simulink model "SPARCS_Mission_System_Composer"  (R2024a)
settings: Solver=VariableStepAuto  StartTime=0.0  StopTime=10.0  RelTol=1e-3
model workspace (MAT data in the model file):
  Communication_Data_Interface = Simulink.Bus
  Communication_Data_Interface.Alignment = -1
  Communication_Data_Interface.PreserveElementDimensions = 0
  Communication_Data_Interface.DataScope = 'Auto'
  Data_Interface = Simulink.Bus
  Data_Interface.Alignment = -1
  Data_Interface.PreserveElementDimensions = 0
  Data_Interface.DataScope = 'Auto'
  Mechanisem_Interface = Simulink.ConnectionBus
  Mechanisem_Interface.Elements_internal(1) = Simulink.ConnectionElement
  Mechanisem_Interface.Elements_internal(1).Name = 'Material'
  Mechanisem_Interface.Elements_internal(1).Type_internal = 'Connection: <domain name>'
  Mechanisem_Interface.Elements_internal(2) = Simulink.ConnectionElement
  Mechanisem_Interface.Elements_internal(2).Name = 'Inpute_Force'
  Mechanisem_Interface.Elements_internal(2).Type_internal = 'Connection: <domain name>'
  Power_Cable = Simulink.ConnectionBus
  Power_Cable.Elements_internal(1) = Simulink.ConnectionElement
  Power_Cable.Elements_internal(1).Name = 'v5'
  Power_Cable.Elements_internal(1).Type_internal = 'Connection: <domain name>'
  Power_Cable.Elements_internal(2) = Simulink.ConnectionElement
  Power_Cable.Elements_internal(2).Name = 'v33'
  Power_Cable.Elements_internal(2).Type_internal = 'Connection: <domain name>'
  Power_Cable.Elements_internal(3) = Simulink.ConnectionElement
  Power_Cable.Elements_internal(3).Name = 'v12'
  Power_Cable.Elements_internal(3).Type_internal = 'Connection: <domain name>'
  Power_Cable.Elements_internal(4) = Simulink.ConnectionElement
  Power_Cable.Elements_internal(4).Name = 'vUnreg'
  Power_Cable.Elements_internal(4).Type_internal = 'Connection: <domain name>'
  Power_Interface = Simulink.Bus
  Power_Interface.Alignment = -1
  Power_Interface.PreserveElementDimensions = 0
  Power_Interface.Elements_internal(1) = Simulink.BusElement
  Power_Interface.Elements_internal(1).Min_internal = 455
  Power_Interface.Elements_internal(1).DimensionsMode = 'Fixed'
  Power_Interface.Elements_internal(1).SamplingMode = 'Sample based'
  Power_Interface.Elements_internal(1).SampleTime = -1
  Power_Interface.Elements_internal(1).Name = 'InstCurrent'
  Power_Interface.Elements_internal(1).DataType_internal = 'double'
  Power_Interface.Elements_internal(1).Complexity = 'real'
  Power_Interface.Elements_internal(1).Dimensions = 1
  Power_Interface.Elements_internal(2) = Simulink.BusElement
  Power_Interface.Elements_internal(2).DimensionsMode = 'Fixed'
  Power_Interface.Elements_internal(2).SamplingMode = 'Sample based'
  Power_Interface.Elements_internal(2).SampleTime = -1
  Power_Interface.Elements_internal(2).Name = 'InstVoltage'
  Power_Interface.Elements_internal(2).DataType_internal = 'double'
  Power_Interface.Elements_internal(2).Complexity = 'real'
  Power_Interface.Elements_internal(2).Dimensions = 1
  Power_Interface.Elements_internal(3) = Simulink.BusElement
  Power_Interface.Elements_internal(3).DimensionsMode = 'Fixed'
  Power_Interface.Elements_internal(3).SamplingMode = 'Sample based'
  Power_Interface.Elements_internal(3).SampleTime = -1
  Power_Interface.Elements_internal(3).Name = 'BatteryVoltage'
  Power_Interface.Elements_internal(3).DataType_internal = 'double'
  Power_Interface.Elements_internal(3).Complexity = 'real'
  Power_Interface.Elements_internal(3).Dimensions = 1
  Power_Interface.DataScope = 'Auto'
undefined symbols (not defined in the file): ADCS, EPS, OBC, Power, TCS, Temp
(part 1 of 2)
settings Model: Creator=Mosavat  LastModifiedBy=dani
settings OptimizationCC: ReuseModelBlockBuffer=off
settings RTWCC: GPUComputeCapability=3.5

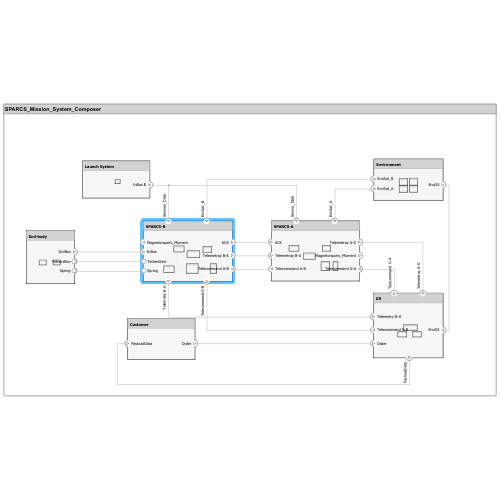
[thumbnail: Simulink's stored preview of the top-level diagram]
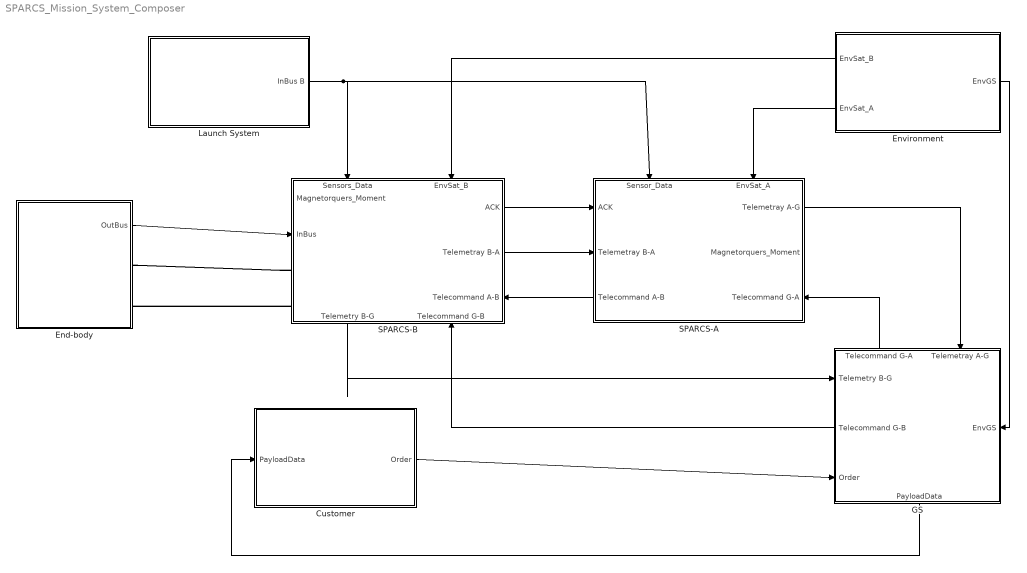
== system SPARCS_Mission_System_Composer ==
  Customer : Subsystem  RequirementInfo={} %GIDa_5276cd9e_2c2d_434b_852c_f5458c074aea
      settings: PortSchema="{\"entries\":[{\"content\":{\"headerSize\":26,\"margin\":15,\"minimumSpacing\":25,\"sides\":[{\"content\":{\"connectorIds\":[\"In1\"]},\"type\":\"ConnectorPlacement.EquallySpacedRectSide\",\"uuid\":\"99c16914-1f21-4030-bd23-0dca739cb4ef\"},{\"content\":{\"connectorIds\":[\"Out1\"],\"side\":\"RIGHT\"},\"type\":\"ConnectorPlacement.EquallySpacedRectSide\",\"uuid\":\"ee0d90fc-8c9e-49ed-bf7b-51fc360639f9\"},{\"content\":{\"connectorIds\":[],\"side\":\"TOP\"},\"type\":\"ConnectorPlacement.EquallySpacedRectSide\",\"uuid\":\"43e54e8f-1cc4-498f-b673-46655361aaba\"}]},\"type\":\"ConnectorPlacement.EquallySpacedConnector\",\"uuid\":\"2a460a3b-dd2b-4c63-a476-f56c55e2bff6\"}],\"packageUris\":[\"http://schema.mathworks.com/mf0/Connector/R2020b\"],\"version\":\"1.0\"}"
  End-body : Subsystem
      settings: PortSchema="{\"entries\":[{\"content\":{\"headerSize\":26,\"margin\":15,\"minimumSpacing\":25,\"sides\":[{\"content\":{\"connectorIds\":[]},\"type\":\"ConnectorPlacement.EquallySpacedRectSide\",\"uuid\":\"e9a48b2f-fbc4-402d-8d97-df232b09ca74\"},{\"content\":{\"connectorIds\":[\"Out1\",\"RConn1\",\"RConn2\"],\"side\":\"RIGHT\"},\"type\":\"ConnectorPlacement.EquallySpacedRectSide\",\"uuid\":\"668a9a5e-c59a-482e-88a8-af4c8ec5a9f3\"},{\"content\":{\"connectorIds\":[],\"side\":\"TOP\"},\"type\":\"ConnectorPlacement.EquallySpacedRectSide\",\"uuid\":\"7c7fce8b-f648-49b4-9dc1-b61d0240baf7\"}]},\"type\":\"ConnectorPlacement.EquallySpacedConnector\",\"uuid\":\"1f193ebe-c506-4262-ad28-c863fe0100e9\"}],\"packageUris\":[\"http://schema.mathworks.com/mf0/Connector/R2020b\"],\"version\":\"1.0\"}"
  Environment : Subsystem  RequirementInfo={} %GIDa_2c95b2b7_b51e_4aa9_866b_417deecfb3d4
      settings: PortSchema="{\"entries\":[{\"content\":{\"headerSize\":26,\"margin\":15,\"minimumSpacing\":25,\"sides\":[{\"content\":{\"connectorIds\":[\"Out1\",\"Out3\"]},\"type\":\"ConnectorPlacement.EquallySpacedRectSide\",\"uuid\":\"99c16914-1f21-4030-bd23-0dca739cb4ef\"},{\"content\":{\"connectorIds\":[\"Out2\"],\"side\":\"RIGHT\"},\"type\":\"ConnectorPlacement.EquallySpacedRectSide\",\"uuid\":\"ee0d90fc-8c9e-49ed-bf7b-51fc360639f9\"},{\"content\":{\"side\":\"TOP\"},\"type\":\"ConnectorPlacement.EquallySpacedRectSide\",\"uuid\":\"43e54e8f-1cc4-498f-b673-46655361aaba\"},{\"content\":{\"side\":\"BOTTOM\"},\"type\":\"ConnectorPlacement.EquallySpacedRectSide\",\"uuid\":\"c295d207-1cb1-4ab0-ab4a-221cf9a33f8c\"}]},\"type\":\"ConnectorPlacement.EquallySpacedConnector\",\"uuid\":\"2a460a3b-dd2b-4c63-a476-f56c55e2bff6\"}],\"packageUris\":[\"http://schema.mathworks.com/mf0/Connector/R2020b\"],\"version\":\"1.0\"}"
  GS : Subsystem  RequirementInfo={} %GIDa_7f442463_82d1_4b26_b178_1c38fd973034
      settings: PortSchema="{\"entries\":[{\"content\":{\"headerSize\":26,\"margin\":15,\"minimumSpacing\":25,\"sides\":[{\"content\":{\"connectorIds\":[\"In1\",\"Out1\",\"In2\"]},\"type\":\"ConnectorPlacement.EquallySpacedRectSide\",\"uuid\":\"99c16914-1f21-4030-bd23-0dca739cb4ef\"},{\"content\":{\"connectorIds\":[\"In4\"],\"side\":\"RIGHT\"},\"type\":\"ConnectorPlacement.EquallySpacedRectSide\",\"uuid\":\"ee0d90fc-8c9e-49ed-bf7b-51fc360639f9\"},{\"content\":{\"connectorIds\":[\"Out3\",\"In3\"],\"side\":\"TOP\"},\"type\":\"ConnectorPlacement.EquallySpacedRectSide\",\"uuid\":\"43e54e8f-1cc4-498f-b673-46655361aaba\"},{\"content\":{\"connectorIds\":[\"Out2\"],\"side\":\"BOTTOM\"},\"type\":\"ConnectorPlacement.EquallySpacedRectSide\",\"uuid\":\"61113e39-adc5-4e36-8ba9-18f5b15ab978\"}]},\"type\":\"ConnectorPlacement.EquallySpacedConnector\",\"uuid\":\"2a460a3b-dd2b-4c63-a476-f56c55e2bff6\"}],\"packageUris\":[\"http://schema.mathworks.com/mf0/Connector/R2020b\"],\"version\":\"1.0\"}"
  Launch System : Subsystem  RequirementInfo={} %GIDa_9d5cdb3d_6dc4_4d26_bfc5_e8ae113977f2
      settings: PortSchema="{\"entries\":[{\"content\":{\"headerSize\":26,\"margin\":15,\"minimumSpacing\":25,\"sides\":[{\"content\":{\"connectorIds\":[]},\"type\":\"ConnectorPlacement.EquallySpacedRectSide\",\"uuid\":\"0e80917e-0df8-41c9-b4a1-578069d1b510\"},{\"content\":{\"connectorIds\":[\"Out1\"],\"side\":\"RIGHT\"},\"type\":\"ConnectorPlacement.EquallySpacedRectSide\",\"uuid\":\"65f7606d-47df-4668-9c7a-3f7124642eb8\"},{\"content\":{\"connectorIds\":[],\"side\":\"TOP\"},\"type\":\"ConnectorPlacement.EquallySpacedRectSide\",\"uuid\":\"3548d248-01fd-4db2-a2f6-b603deefc062\"}]},\"type\":\"ConnectorPlacement.EquallySpacedConnector\",\"uuid\":\"f365137c-e6cc-4032-bc65-cfd89a070f7f\"}],\"packageUris\":[\"http://schema.mathworks.com/mf0/Connector/R2020b\"],\"version\":\"1.0\"}"
  SPARCS-A : Subsystem  RequirementInfo="{}  %GIDa_bb889290_f2af_4178_93e4_6d667fc14114"
      settings: PortSchema="{\"entries\":[{\"content\":{\"headerSize\":26,\"margin\":15,\"minimumSpacing\":25,\"sides\":[{\"content\":{\"connectorIds\":[\"In1\",\"In2\",\"Out1\"]},\"type\":\"ConnectorPlacement.EquallySpacedRectSide\",\"uuid\":\"e9a48b2f-fbc4-402d-8d97-df232b09ca74\"},{\"content\":{\"connectorIds\":[\"Out3\",\"Out2\",\"In3\"],\"side\":\"RIGHT\"},\"type\":\"ConnectorPlacement.EquallySpacedRectSide\",\"uuid\":\"668a9a5e-c59a-482e-88a8-af4c8ec5a9f3\"},{\"content\":{\"connectorIds\":[\"In4\",\"In5\"],\"side\":\"TOP\"},\"type\":\"ConnectorPlacement.EquallySpacedRectSide\",\"uuid\":\"7c7fce8b-f648-49b4-9dc1-b61d0240baf7\"}]},\"type\":\"ConnectorPlacement.EquallySpacedConnector\",\"uuid\":\"1f193ebe-c506-4262-ad28-c863fe0100e9\"}],\"packageUris\":[\"http://schema.mathworks.com/mf0/Connector/R2020b\"],\"version\":\"1.0\"}"
  SPARCS-B : Subsystem
      settings: PortSchema="{\"entries\":[{\"content\":{\"headerSize\":26,\"margin\":15,\"minimumSpacing\":25,\"sides\":[{\"content\":{\"connectorIds\":[\"Out3\",\"In3\",\"LConn1\",\"LConn2\"]},\"type\":\"ConnectorPlacement.EquallySpacedRectSide\",\"uuid\":\"e9a48b2f-fbc4-402d-8d97-df232b09ca74\"},{\"content\":{\"connectorIds\":[\"Out2\",\"Out4\",\"In4\"],\"side\":\"RIGHT\"},\"type\":\"ConnectorPlacement.EquallySpacedRectSide\",\"uuid\":\"668a9a5e-c59a-482e-88a8-af4c8ec5a9f3\"},{\"content\":{\"connectorIds\":[\"In5\",\"In2\"],\"side\":\"TOP\"},\"type\":\"ConnectorPlacement.EquallySpacedRectSide\",\"uuid\":\"7c7fce8b-f648-49b4-9dc1-b61d0240baf7\"},{\"content\":{\"connectorIds\":[\"Out1\",\"In1\"],\"side\":\"BOTTOM\"},\"type\":\"ConnectorPlacement.EquallySpacedRectSide\",\"uuid\":\"24f8add0-5994-41fc-ad83-a43d4515e3f5\"}]},\"type\":\"ConnectorPlacement.EquallySpacedConnector\",\"uuid\":\"1f193ebe-c506-4262-ad28-c863fe0100e9\"}],\"packageUris\":[\"http://schema.mathworks.com/mf0/Connector/R2020b\"],\"version\":\"1.0\"}"
  wires:
  Launch System/1(InBus B) -> SPARCS-A/4(Sensor_Data), SPARCS-B/5(Sensors_Data)
  Environment/3(EnvSat_A) -> SPARCS-A/5(EnvSat_A)
  Environment/2(EnvGS) -> GS/4(EnvGS)
  GS/3(Telecommand G-A) -> SPARCS-A/3(Telecommand G-A)
  SPARCS-A/3(Telemetray A-G) -> GS/3(Telemetray A-G)
  Customer/1(Order) -> GS/2(Order)
  GS/2(PayloadData) -> Customer/1(PayloadData)
  SPARCS-B/4(Telemetray B-A) -> SPARCS-A/2(Telemetray B-A)
  SPARCS-A/1(Telecommand A-B) -> SPARCS-B/4(Telecommand A-B)
  End-body/1(OutBus) -> SPARCS-B/3(InBus)
  SPARCS-B/2(ACK) -> SPARCS-A/1(ACK)
  SPARCS-B/1(Telemetry B-G) -> GS/1(Telemetry B-G)
  GS/1(Telecommand G-B) -> SPARCS-B/1(Telecommand G-B)
  Environment/1(EnvSat_B) -> SPARCS-B/2(EnvSat_B)
  connections:
  SPARCS-B/LConn1 -- End-body/RConn1
  SPARCS-B/LConn2 -- End-body/RConn2

== system SPARCS_Mission_System_Composer/Customer ==
  Bus Element In1 : Inport  RequirementInfo={} %GIDa_50217abe_56c4_45ce_a731_87f8e4f342ac  PortName=PayloadData
  Bus Element Out1 : Outport  RequirementInfo={} %GIDa_63cfd474_b787_456e_9731_ad5e1ed17cae  PortName=Order

== system SPARCS_Mission_System_Composer/End-body ==
  Collector : Subsystem
      settings: PortSchema="{\"entries\":[{\"content\":{\"headerSize\":26,\"margin\":15,\"minimumSpacing\":25,\"sides\":[{\"content\":{\"connectorIds\":[]},\"type\":\"ConnectorPlacement.EquallySpacedRectSide\",\"uuid\":\"b0f3186e-f576-4647-b1a2-44485358b727\"},{\"content\":{\"connectorIds\":[],\"side\":\"RIGHT\"},\"type\":\"ConnectorPlacement.EquallySpacedRectSide\",\"uuid\":\"71064ded-3aa0-4a06-beed-3d1d2c210288\"},{\"content\":{\"connectorIds\":[],\"side\":\"TOP\"},\"type\":\"ConnectorPlacement.EquallySpacedRectSide\",\"uuid\":\"7b8a25e8-1259-40c4-b5f8-7d1b8fa69d47\"}]},\"type\":\"ConnectorPlacement.EquallySpacedConnector\",\"uuid\":\"e60708fb-7212-4361-80b1-30af05aaea9b\"}],\"packageUris\":[\"http://schema.mathworks.com/mf0/Connector/R2020b\"],\"version\":\"1.0\"}"
  Emitter : Subsystem
      settings: PortSchema="{\"entries\":[{\"content\":{\"headerSize\":26,\"margin\":15,\"minimumSpacing\":25,\"sides\":[{\"content\":{\"connectorIds\":[]},\"type\":\"ConnectorPlacement.EquallySpacedRectSide\",\"uuid\":\"b0f3186e-f576-4647-b1a2-44485358b727\"},{\"content\":{\"connectorIds\":[],\"side\":\"RIGHT\"},\"type\":\"ConnectorPlacement.EquallySpacedRectSide\",\"uuid\":\"71064ded-3aa0-4a06-beed-3d1d2c210288\"},{\"content\":{\"connectorIds\":[],\"side\":\"TOP\"},\"type\":\"ConnectorPlacement.EquallySpacedRectSide\",\"uuid\":\"7b8a25e8-1259-40c4-b5f8-7d1b8fa69d47\"}]},\"type\":\"ConnectorPlacement.EquallySpacedConnector\",\"uuid\":\"e60708fb-7212-4361-80b1-30af05aaea9b\"}],\"packageUris\":[\"http://schema.mathworks.com/mf0/Connector/R2020b\"],\"version\":\"1.0\"}"
  TetherWire : PMIOPort  Side=Right
  Spring : PMIOPort  Port=2  Side=Right
  Bus Element Out1 : Outport  PortName=OutBus

== system SPARCS_Mission_System_Composer/Environment ==
  Atmosphere : Subsystem  RequirementInfo={} %GIDa_eb05b99d_c241_4e54_a779_761c9347d3e2
      settings: PortSchema="{\"entries\":[{\"content\":{\"headerSize\":26,\"margin\":15,\"minimumSpacing\":25,\"sides\":[{\"content\":{\"connectorIds\":[]},\"type\":\"ConnectorPlacement.EquallySpacedRectSide\",\"uuid\":\"a0205618-f388-4a93-9aec-aa689e4ebd78\"},{\"content\":{\"connectorIds\":[],\"side\":\"RIGHT\"},\"type\":\"ConnectorPlacement.EquallySpacedRectSide\",\"uuid\":\"79acb52b-c683-45c4-8f19-6aa7b44b6a95\"},{\"content\":{\"connectorIds\":[],\"side\":\"TOP\"},\"type\":\"ConnectorPlacement.EquallySpacedRectSide\",\"uuid\":\"1a3a54da-b4f5-4a0e-9102-49590a789f5c\"}]},\"type\":\"ConnectorPlacement.EquallySpacedConnector\",\"uuid\":\"e5b731ae-b390-48dd-b7a1-3459e2e6bab0\"}],\"packageUris\":[\"http://schema.mathworks.com/mf0/Connector/R2020b\"],\"version\":\"1.0\"}"
  Earth : Subsystem  RequirementInfo={} %GIDa_b95c931a_ef81_4893_b6c0_be75a463d49e
      settings: PortSchema="{\"entries\":[{\"content\":{\"headerSize\":26,\"margin\":15,\"minimumSpacing\":25,\"sides\":[{\"content\":{\"connectorIds\":[]},\"type\":\"ConnectorPlacement.EquallySpacedRectSide\",\"uuid\":\"a0205618-f388-4a93-9aec-aa689e4ebd78\"},{\"content\":{\"connectorIds\":[],\"side\":\"RIGHT\"},\"type\":\"ConnectorPlacement.EquallySpacedRectSide\",\"uuid\":\"79acb52b-c683-45c4-8f19-6aa7b44b6a95\"},{\"content\":{\"connectorIds\":[],\"side\":\"TOP\"},\"type\":\"ConnectorPlacement.EquallySpacedRectSide\",\"uuid\":\"1a3a54da-b4f5-4a0e-9102-49590a789f5c\"}]},\"type\":\"ConnectorPlacement.EquallySpacedConnector\",\"uuid\":\"e5b731ae-b390-48dd-b7a1-3459e2e6bab0\"}],\"packageUris\":[\"http://schema.mathworks.com/mf0/Connector/R2020b\"],\"version\":\"1.0\"}"
  Sun : Subsystem  RequirementInfo={} %GIDa_99381c14_de20_4199_bf05_b451084bd8b9
      settings: PortSchema="{\"entries\":[{\"content\":{\"headerSize\":26,\"margin\":15,\"minimumSpacing\":25,\"sides\":[{\"content\":{\"connectorIds\":[]},\"type\":\"ConnectorPlacement.EquallySpacedRectSide\",\"uuid\":\"a0205618-f388-4a93-9aec-aa689e4ebd78\"},{\"content\":{\"connectorIds\":[],\"side\":\"RIGHT\"},\"type\":\"ConnectorPlacement.EquallySpacedRectSide\",\"uuid\":\"79acb52b-c683-45c4-8f19-6aa7b44b6a95\"},{\"content\":{\"connectorIds\":[],\"side\":\"TOP\"},\"type\":\"ConnectorPlacement.EquallySpacedRectSide\",\"uuid\":\"1a3a54da-b4f5-4a0e-9102-49590a789f5c\"}]},\"type\":\"ConnectorPlacement.EquallySpacedConnector\",\"uuid\":\"e5b731ae-b390-48dd-b7a1-3459e2e6bab0\"}],\"packageUris\":[\"http://schema.mathworks.com/mf0/Connector/R2020b\"],\"version\":\"1.0\"}"
  Time : Subsystem  RequirementInfo={} %GIDa_8bde8406_355b_4db9_a468_32211b2e0ea2
      settings: PortSchema="{\"entries\":[{\"content\":{\"headerSize\":26,\"margin\":15,\"minimumSpacing\":25,\"sides\":[{\"content\":{\"connectorIds\":[]},\"type\":\"ConnectorPlacement.EquallySpacedRectSide\",\"uuid\":\"a0205618-f388-4a93-9aec-aa689e4ebd78\"},{\"content\":{\"connectorIds\":[],\"side\":\"RIGHT\"},\"type\":\"ConnectorPlacement.EquallySpacedRectSide\",\"uuid\":\"79acb52b-c683-45c4-8f19-6aa7b44b6a95\"},{\"content\":{\"connectorIds\":[],\"side\":\"TOP\"},\"type\":\"ConnectorPlacement.EquallySpacedRectSide\",\"uuid\":\"1a3a54da-b4f5-4a0e-9102-49590a789f5c\"}]},\"type\":\"ConnectorPlacement.EquallySpacedConnector\",\"uuid\":\"e5b731ae-b390-48dd-b7a1-3459e2e6bab0\"}],\"packageUris\":[\"http://schema.mathworks.com/mf0/Connector/R2020b\"],\"version\":\"1.0\"}"
  Bus Element Out3 : Outport  PortName=EnvSat_B
  Bus Element Out2 : Outport  RequirementInfo={} %GIDa_4f6e6d30_9ff6_4620_aadf_7d15cb6fc292  Port=2  PortName=EnvGS
  Bus Element Out1 : Outport  RequirementInfo={} %GIDa_ad4902e5_7a7f_4265_b3dc_3808822d8108  Port=3  PortName=EnvSat_A

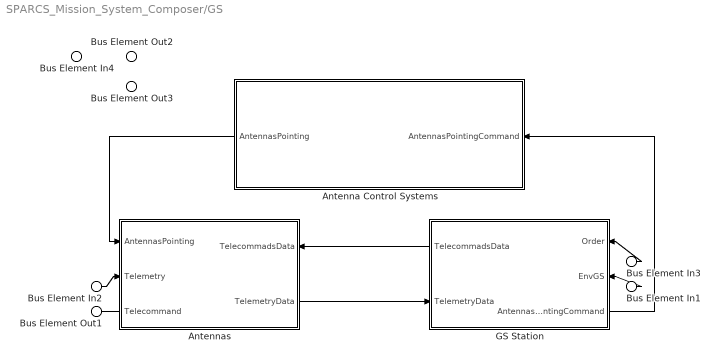
== system SPARCS_Mission_System_Composer/GS ==
  Bus Element In4 : Inport  PortName=Telemetry B-G
  Bus Element In3 : Inport  RequirementInfo={} %GIDa_1c5e6e98_e2f6_49b9_9cfa_88040fc1fba5  Port=2  PortName=Order
  Bus Element In2 : Inport  RequirementInfo={} %GIDa_0c79b00d_9eca_49d8_adcc_d17375f08e84  Port=3  PortName=Telemetray A-G
  Bus Element In1 : Inport  RequirementInfo={} %GIDa_ac8f2bba_56c0_4e78_a408_5eec346da907  Port=4  PortName=EnvGS
  Antenna Control Systems : Subsystem  RequirementInfo={} %GIDa_89f6fcc8_7c51_47bb_b8d5_8a1504126ec7
      settings: PortSchema="{\"entries\":[{\"content\":{\"headerSize\":26,\"margin\":15,\"minimumSpacing\":25,\"sides\":[{\"content\":{\"connectorIds\":[\"Out1\"]},\"type\":\"ConnectorPlacement.EquallySpacedRectSide\",\"uuid\":\"a0205618-f388-4a93-9aec-aa689e4ebd78\"},{\"content\":{\"connectorIds\":[\"In1\"],\"side\":\"RIGHT\"},\"type\":\"ConnectorPlacement.EquallySpacedRectSide\",\"uuid\":\"79acb52b-c683-45c4-8f19-6aa7b44b6a95\"},{\"content\":{\"connectorIds\":[],\"side\":\"TOP\"},\"type\":\"ConnectorPlacement.EquallySpacedRectSide\",\"uuid\":\"1a3a54da-b4f5-4a0e-9102-49590a789f5c\"},{\"content\":{\"connectorIds\":[],\"side\":\"BOTTOM\"},\"type\":\"ConnectorPlacement.EquallySpacedRectSide\",\"uuid\":\"9ac2cda3-0247-4f52-b572-2154d037acfc\"}]},\"type\":\"ConnectorPlacement.EquallySpacedConnector\",\"uuid\":\"e5b731ae-b390-48dd-b7a1-3459e2e6bab0\"}],\"packageUris\":[\"http://schema.mathworks.com/mf0/Connector/R2020b\"],\"version\":\"1.0\"}"
  Antennas : Subsystem  RequirementInfo={} %GIDa_95957288_8d11_42dc_b667_82305f244e57
      settings: PortSchema="{\"entries\":[{\"content\":{\"headerSize\":26,\"margin\":15,\"minimumSpacing\":25,\"sides\":[{\"content\":{\"connectorIds\":[\"In2\",\"In3\",\"Out2\"]},\"type\":\"ConnectorPlacement.EquallySpacedRectSide\",\"uuid\":\"a0205618-f388-4a93-9aec-aa689e4ebd78\"},{\"content\":{\"connectorIds\":[\"In1\",\"Out1\"],\"side\":\"RIGHT\"},\"type\":\"ConnectorPlacement.EquallySpacedRectSide\",\"uuid\":\"79acb52b-c683-45c4-8f19-6aa7b44b6a95\"},{\"content\":{\"connectorIds\":[],\"side\":\"TOP\"},\"type\":\"ConnectorPlacement.EquallySpacedRectSide\",\"uuid\":\"1a3a54da-b4f5-4a0e-9102-49590a789f5c\"}]},\"type\":\"ConnectorPlacement.EquallySpacedConnector\",\"uuid\":\"e5b731ae-b390-48dd-b7a1-3459e2e6bab0\"}],\"packageUris\":[\"http://schema.mathworks.com/mf0/Connector/R2020b\"],\"version\":\"1.0\"}"
  GS Station : Subsystem  RequirementInfo={} %GIDa_50bc68e1_b1a0_408f_93ec_e9ab810c3ebe
      settings: PortSchema="{\"entries\":[{\"content\":{\"headerSize\":26,\"margin\":15,\"minimumSpacing\":25,\"sides\":[{\"content\":{\"connectorIds\":[\"Out1\",\"In3\"]},\"type\":\"ConnectorPlacement.EquallySpacedRectSide\",\"uuid\":\"a0205618-f388-4a93-9aec-aa689e4ebd78\"},{\"content\":{\"connectorIds\":[\"In1\",\"In2\",\"Out2\"],\"side\":\"RIGHT\"},\"type\":\"ConnectorPlacement.EquallySpacedRectSide\",\"uuid\":\"79acb52b-c683-45c4-8f19-6aa7b44b6a95\"},{\"content\":{\"connectorIds\":[],\"side\":\"TOP\"},\"type\":\"ConnectorPlacement.EquallySpacedRectSide\",\"uuid\":\"1a3a54da-b4f5-4a0e-9102-49590a789f5c\"},{\"content\":{\"connectorIds\":[],\"side\":\"BOTTOM\"},\"type\":\"ConnectorPlacement.EquallySpacedRectSide\",\"uuid\":\"a0883a5f-cb12-4437-b239-442920e299fa\"}]},\"type\":\"ConnectorPlacement.EquallySpacedConnector\",\"uuid\":\"e5b731ae-b390-48dd-b7a1-3459e2e6bab0\"}],\"packageUris\":[\"http://schema.mathworks.com/mf0/Connector/R2020b\"],\"version\":\"1.0\"}"
  Bus Element Out3 : Outport  PortName=Telecommand G-B
  Bus Element Out2 : Outport  Port=2  PortName=PayloadData
  Bus Element Out1 : Outport  RequirementInfo={} %GIDa_51763359_9ab6_48ad_b447_d543d03ee004  Port=3  PortName=Telecommand G-A
  wires:
  Bus Element In2/1 -> Antennas/3(Telemetry)
  Antennas/2(Telecommand) -> Bus Element Out1/1
  Antenna Control Systems/1(AntennasPointing) -> Antennas/2(AntennasPointing)
  GS Station/2(AntennasPointingCommand) -> Antenna Control Systems/1(AntennasPointingCommand)
  GS Station/1(TelecommadsData) -> Antennas/1(TelecommadsData)
  Antennas/1(TelemetryData) -> GS Station/3(TelemetryData)
  Bus Element In1/1 -> GS Station/2(EnvGS)
  Bus Element In3/1 -> GS Station/1(Order)

== system SPARCS_Mission_System_Composer/Launch System ==
  Component : Subsystem
      settings: PortSchema="{\"entries\":[{\"content\":{\"headerSize\":26,\"margin\":15,\"minimumSpacing\":25,\"sides\":[{\"content\":{\"connectorIds\":[]},\"type\":\"ConnectorPlacement.EquallySpacedRectSide\",\"uuid\":\"9a7037ce-e1a5-4d46-8111-5886fddb9b24\"},{\"content\":{\"connectorIds\":[],\"side\":\"RIGHT\"},\"type\":\"ConnectorPlacement.EquallySpacedRectSide\",\"uuid\":\"20b2048c-0904-414d-8c49-ea2b529604ef\"},{\"content\":{\"connectorIds\":[],\"side\":\"TOP\"},\"type\":\"ConnectorPlacement.EquallySpacedRectSide\",\"uuid\":\"32c6da6e-71f7-4ed5-82cb-cf1b28c2bdf7\"}]},\"type\":\"ConnectorPlacement.EquallySpacedConnector\",\"uuid\":\"f6c8ad2c-3d58-4ab6-b863-3f028749c78d\"}],\"packageUris\":[\"http://schema.mathworks.com/mf0/Connector/R2020b\"],\"version\":\"1.0\"}"
  Bus Element Out1 : Outport  RequirementInfo={} %GIDa_f2808e3f_afc6_412a_b6c0_e64b71cecebd  PortName=InBus B

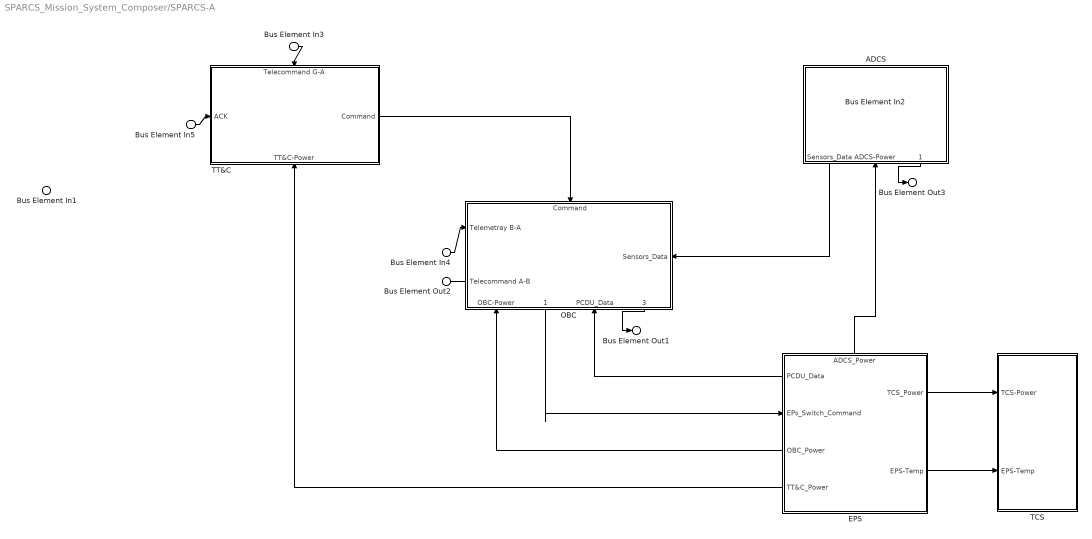
== system SPARCS_Mission_System_Composer/SPARCS-A ==
  Bus Element In5 : Inport  PortName=ACK
  Bus Element In4 : Inport  Port=2  PortName=Telemetray B-A
  Bus Element In3 : Inport  Port=3  PortName=Telecommand G-A
  Bus Element In1 : Inport  Port=4  PortName=Sensor_Data
  Bus Element In2 : Inport  Port=5  PortName=EnvSat_A
  ADCS : Subsystem
      settings: PortSchema="{\"entries\":[{\"content\":{\"headerSize\":26,\"margin\":15,\"minimumSpacing\":25,\"sides\":[{\"content\":{\"connectorIds\":[]},\"type\":\"ConnectorPlacement.EquallySpacedRectSide\",\"uuid\":\"e9a48b2f-fbc4-402d-8d97-df232b09ca74\"},{\"content\":{\"connectorIds\":[],\"side\":\"RIGHT\"},\"type\":\"ConnectorPlacement.EquallySpacedRectSide\",\"uuid\":\"668a9a5e-c59a-482e-88a8-af4c8ec5a9f3\"},{\"content\":{\"connectorIds\":[],\"side\":\"TOP\"},\"type\":\"ConnectorPlacement.EquallySpacedRectSide\",\"uuid\":\"7c7fce8b-f648-49b4-9dc1-b61d0240baf7\"},{\"content\":{\"connectorIds\":[\"Out2\",\"In1\",\"Out1\"],\"side\":\"BOTTOM\"},\"type\":\"ConnectorPlacement.EquallySpacedRectSide\",\"uuid\":\"2c3f5986-9b39-4ef3-b054-4f041a587ca4\"}]},\"type\":\"ConnectorPlacement.EquallySpacedConnector\",\"uuid\":\"1f193ebe-c506-4262-ad28-c863fe0100e9\"}],\"packageUris\":[\"http://schema.mathworks.com/mf0/Connector/R2020b\"],\"version\":\"1.0\"}"
  EPS : Subsystem
      settings: PortSchema="{\"entries\":[{\"content\":{\"headerSize\":26,\"margin\":15,\"minimumSpacing\":25,\"sides\":[{\"content\":{\"connectorIds\":[\"Out1\",\"In1\",\"Out5\",\"Out6\"]},\"type\":\"ConnectorPlacement.EquallySpacedRectSide\",\"uuid\":\"e9a48b2f-fbc4-402d-8d97-df232b09ca74\"},{\"content\":{\"connectorIds\":[\"Out2\",\"Out3\"],\"side\":\"RIGHT\"},\"type\":\"ConnectorPlacement.EquallySpacedRectSide\",\"uuid\":\"668a9a5e-c59a-482e-88a8-af4c8ec5a9f3\"},{\"content\":{\"connectorIds\":[\"Out4\"],\"side\":\"TOP\"},\"type\":\"ConnectorPlacement.EquallySpacedRectSide\",\"uuid\":\"7c7fce8b-f648-49b4-9dc1-b61d0240baf7\"},{\"content\":{\"connectorIds\":[],\"side\":\"BOTTOM\"},\"type\":\"ConnectorPlacement.EquallySpacedRectSide\",\"uuid\":\"3e521869-eeda-4ec5-bb7d-2b348f8e7054\"}]},\"type\":\"ConnectorPlacement.EquallySpacedConnector\",\"uuid\":\"1f193ebe-c506-4262-ad28-c863fe0100e9\"}],\"packageUris\":[\"http://schema.mathworks.com/mf0/Connector/R2020b\"],\"version\":\"1.0\"}"
  OBC : Subsystem
      settings: PortSchema="{\"entries\":[{\"content\":{\"headerSize\":26,\"margin\":15,\"minimumSpacing\":25,\"sides\":[{\"content\":{\"connectorIds\":[\"In3\",\"Out2\"]},\"type\":\"ConnectorPlacement.EquallySpacedRectSide\",\"uuid\":\"e9a48b2f-fbc4-402d-8d97-df232b09ca74\"},{\"content\":{\"connectorIds\":[\"In4\"],\"side\":\"RIGHT\"},\"type\":\"ConnectorPlacement.EquallySpacedRectSide\",\"uuid\":\"668a9a5e-c59a-482e-88a8-af4c8ec5a9f3\"},{\"content\":{\"connectorIds\":[\"In1\"],\"side\":\"TOP\"},\"type\":\"ConnectorPlacement.EquallySpacedRectSide\",\"uuid\":\"7c7fce8b-f648-49b4-9dc1-b61d0240baf7\"},{\"content\":{\"connectorIds\":[\"In5\",\"Out1\",\"In2\",\"Out3\"],\"side\":\"BOTTOM\"},\"type\":\"ConnectorPlacement.EquallySpacedRectSide\",\"uuid\":\"b1c700a7-d344-470e-b338-9b978c458512\"}]},\"type\":\"ConnectorPlacement.EquallySpacedConnector\",\"uuid\":\"1f193ebe-c506-4262-ad28-c863fe0100e9\"}],\"packageUris\":[\"http://schema.mathworks.com/mf0/Connector/R2020b\"],\"version\":\"1.0\"}"
  TCS : Subsystem
      settings: PortSchema="{\"entries\":[{\"content\":{\"headerSize\":26,\"margin\":15,\"minimumSpacing\":25,\"sides\":[{\"content\":{\"connectorIds\":[\"In2\",\"In1\"]},\"type\":\"ConnectorPlacement.EquallySpacedRectSide\",\"uuid\":\"e9a48b2f-fbc4-402d-8d97-df232b09ca74\"},{\"content\":{\"connectorIds\":[],\"side\":\"RIGHT\"},\"type\":\"ConnectorPlacement.EquallySpacedRectSide\",\"uuid\":\"668a9a5e-c59a-482e-88a8-af4c8ec5a9f3\"},{\"content\":{\"connectorIds\":[],\"side\":\"TOP\"},\"type\":\"ConnectorPlacement.EquallySpacedRectSide\",\"uuid\":\"7c7fce8b-f648-49b4-9dc1-b61d0240baf7\"},{\"content\":{\"connectorIds\":[],\"side\":\"BOTTOM\"},\"type\":\"ConnectorPlacement.EquallySpacedRectSide\",\"uuid\":\"b0f76e66-ab31-4e75-aed3-a16376b57c27\"}]},\"type\":\"ConnectorPlacement.EquallySpacedConnector\",\"uuid\":\"1f193ebe-c506-4262-ad28-c863fe0100e9\"}],\"packageUris\":[\"http://schema.mathworks.com/mf0/Connector/R2020b\"],\"version\":\"1.0\"}"
  "TT&C " : Subsystem
      settings: PortSchema="{\"entries\":[{\"content\":{\"headerSize\":26,\"margin\":15,\"minimumSpacing\":25,\"sides\":[{\"content\":{\"connectorIds\":[\"In1\"]},\"type\":\"ConnectorPlacement.EquallySpacedRectSide\",\"uuid\":\"e9a48b2f-fbc4-402d-8d97-df232b09ca74\"},{\"content\":{\"connectorIds\":[\"Out1\"],\"side\":\"RIGHT\"},\"type\":\"ConnectorPlacement.EquallySpacedRectSide\",\"uuid\":\"668a9a5e-c59a-482e-88a8-af4c8ec5a9f3\"},{\"content\":{\"connectorIds\":[\"In2\"],\"side\":\"TOP\"},\"type\":\"ConnectorPlacement.EquallySpacedRectSide\",\"uuid\":\"7c7fce8b-f648-49b4-9dc1-b61d0240baf7\"},{\"content\":{\"connectorIds\":[\"In3\"],\"side\":\"BOTTOM\"},\"type\":\"ConnectorPlacement.EquallySpacedRectSide\",\"uuid\":\"48187e99-04ba-46d1-bed4-4c5e9e3f3fd7\"}]},\"type\":\"ConnectorPlacement.EquallySpacedConnector\",\"uuid\":\"1f193ebe-c506-4262-ad28-c863fe0100e9\"}],\"packageUris\":[\"http://schema.mathworks.com/mf0/Connector/R2020b\"],\"version\":\"1.0\"}"
  Bus Element Out2 : Outport  PortName=Telecommand A-B
  Bus Element Out3 : Outport  Port=2  PortName=Magnetorquers_Moment
  Bus Element Out1 : Outport  Port=3  PortName=Telemetray A-G
  wires:
  EPS/6(TT&C_Power) -> "TT&C "/3(TT&C-Power)
  EPS/5(OBC_Power) -> OBC/5(OBC-Power)
  EPS/4(ADCS_Power) -> ADCS/1(ADCS-Power)
  ADCS/2(Sensors_Data) -> OBC/4(Sensors_Data)
  EPS/2(TCS_Power) -> TCS/2(TCS-Power)
  EPS/3(EPS-Temp) -> TCS/1(EPS-Temp)
  Bus Element In3/1 -> "TT&C "/2(Telecommand G-A)
  Bus Element In5/1 -> "TT&C "/1(ACK)
  OBC/3(Telemetray A-G) -> Bus Element Out1/1
  ADCS/1(Magnetorquers_Moment) -> Bus Element Out3/1
  Bus Element In4/1 -> OBC/3(Telemetray B-A)
  OBC/2(Telecommand A-B) -> Bus Element Out2/1
  "TT&C "/1(Command) -> OBC/1(Command)
  EPS/1(PCDU_Data) -> OBC/2(PCDU_Data)
  OBC/1(EPs_Switch_Command) -> EPS/1(EPs_Switch_Command)

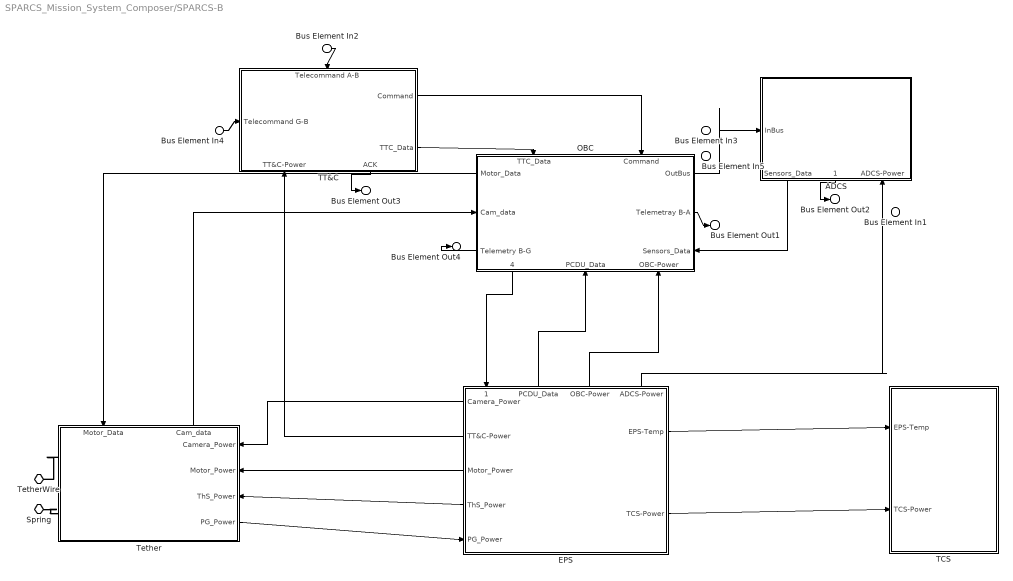
== system SPARCS_Mission_System_Composer/SPARCS-B ==
  Bus Element In4 : Inport  PortName=Telecommand G-B
  Bus Element In5 : Inport  Port=2  PortName=EnvSat_B
  Bus Element In3 : Inport  Port=3  PortName=InBus
  Bus Element In2 : Inport  Port=4  PortName=Telecommand A-B
  Bus Element In1 : Inport  Port=5  PortName=Sensors_Data
  ADCS : Subsystem
      settings: PortSchema="{\"entries\":[{\"content\":{\"headerSize\":26,\"margin\":15,\"minimumSpacing\":25,\"sides\":[{\"content\":{\"connectorIds\":[\"In1\"]},\"type\":\"ConnectorPlacement.EquallySpacedRectSide\",\"uuid\":\"e9a48b2f-fbc4-402d-8d97-df232b09ca74\"},{\"content\":{\"side\":\"RIGHT\"},\"type\":\"ConnectorPlacement.EquallySpacedRectSide\",\"uuid\":\"668a9a5e-c59a-482e-88a8-af4c8ec5a9f3\"},{\"content\":{\"side\":\"TOP\"},\"type\":\"ConnectorPlacement.EquallySpacedRectSide\",\"uuid\":\"7c7fce8b-f648-49b4-9dc1-b61d0240baf7\"},{\"content\":{\"connectorIds\":[\"Out2\",\"Out1\",\"In2\"],\"side\":\"BOTTOM\"},\"type\":\"ConnectorPlacement.EquallySpacedRectSide\",\"uuid\":\"2c3f5986-9b39-4ef3-b054-4f041a587ca4\"}]},\"type\":\"ConnectorPlacement.EquallySpacedConnector\",\"uuid\":\"1f193ebe-c506-4262-ad28-c863fe0100e9\"}],\"packageUris\":[\"http://schema.mathworks.com/mf0/Connector/R2020b\"],\"version\":\"1.0\"}"
  EPS : Subsystem
      settings: PortSchema="{\"entries\":[{\"content\":{\"headerSize\":26,\"margin\":15,\"minimumSpacing\":25,\"sides\":[{\"content\":{\"connectorIds\":[\"Out1\",\"Out9\",\"Out3\",\"Out5\",\"In2\"]},\"type\":\"ConnectorPlacement.EquallySpacedRectSide\",\"uuid\":\"e9a48b2f-fbc4-402d-8d97-df232b09ca74\"},{\"content\":{\"connectorIds\":[\"Out6\",\"Out4\"],\"side\":\"RIGHT\"},\"type\":\"ConnectorPlacement.EquallySpacedRectSide\",\"uuid\":\"668a9a5e-c59a-482e-88a8-af4c8ec5a9f3\"},{\"content\":{\"connectorIds\":[\"In1\",\"Out2\",\"Out8\",\"Out7\"],\"side\":\"TOP\"},\"type\":\"ConnectorPlacement.EquallySpacedRectSide\",\"uuid\":\"7c7fce8b-f648-49b4-9dc1-b61d0240baf7\"},{\"content\":{\"connectorIds\":[],\"side\":\"BOTTOM\"},\"type\":\"ConnectorPlacement.EquallySpacedRectSide\",\"uuid\":\"3e521869-eeda-4ec5-bb7d-2b348f8e7054\"}]},\"type\":\"ConnectorPlacement.EquallySpacedConnector\",\"uuid\":\"1f193ebe-c506-4262-ad28-c863fe0100e9\"}],\"packageUris\":[\"http://schema.mathworks.com/mf0/Connector/R2020b\"],\"version\":\"1.0\"}"
  OBC : Subsystem
      settings: PortSchema="{\"entries\":[{\"content\":{\"headerSize\":26,\"margin\":15,\"minimumSpacing\":25,\"sides\":[{\"content\":{\"connectorIds\":[\"Out5\",\"In4\",\"Out2\"]},\"type\":\"ConnectorPlacement.EquallySpacedRectSide\",\"uuid\":\"e9a48b2f-fbc4-402d-8d97-df232b09ca74\"},{\"content\":{\"connectorIds\":[\"Out1\",\"Out3\",\"In5\"],\"side\":\"RIGHT\"},\"type\":\"ConnectorPlacement.EquallySpacedRectSide\",\"uuid\":\"668a9a5e-c59a-482e-88a8-af4c8ec5a9f3\"},{\"content\":{\"connectorIds\":[\"In1\",\"In3\"],\"side\":\"TOP\"},\"type\":\"ConnectorPlacement.EquallySpacedRectSide\",\"uuid\":\"7c7fce8b-f648-49b4-9dc1-b61d0240baf7\"},{\"content\":{\"connectorIds\":[\"Out4\",\"In2\",\"In6\"],\"side\":\"BOTTOM\"},\"type\":\"ConnectorPlacement.EquallySpacedRectSide\",\"uuid\":\"b1c700a7-d344-470e-b338-9b978c458512\"}]},\"type\":\"ConnectorPlacement.EquallySpacedConnector\",\"uuid\":\"1f193ebe-c506-4262-ad28-c863fe0100e9\"}],\"packageUris\":[\"http://schema.mathworks.com/mf0/Connector/R2020b\"],\"version\":\"1.0\"}"
  TCS : Subsystem
      settings: PortSchema="{\"entries\":[{\"content\":{\"headerSize\":26,\"margin\":15,\"minimumSpacing\":25,\"sides\":[{\"content\":{\"connectorIds\":[\"In1\",\"In2\"]},\"type\":\"ConnectorPlacement.EquallySpacedRectSide\",\"uuid\":\"e9a48b2f-fbc4-402d-8d97-df232b09ca74\"},{\"content\":{\"connectorIds\":[],\"side\":\"RIGHT\"},\"type\":\"ConnectorPlacement.EquallySpacedRectSide\",\"uuid\":\"668a9a5e-c59a-482e-88a8-af4c8ec5a9f3\"},{\"content\":{\"connectorIds\":[],\"side\":\"TOP\"},\"type\":\"ConnectorPlacement.EquallySpacedRectSide\",\"uuid\":\"7c7fce8b-f648-49b4-9dc1-b61d0240baf7\"},{\"content\":{\"connectorIds\":[],\"side\":\"BOTTOM\"},\"type\":\"ConnectorPlacement.EquallySpacedRectSide\",\"uuid\":\"b0f76e66-ab31-4e75-aed3-a16376b57c27\"}]},\"type\":\"ConnectorPlacement.EquallySpacedConnector\",\"uuid\":\"1f193ebe-c506-4262-ad28-c863fe0100e9\"}],\"packageUris\":[\"http://schema.mathworks.com/mf0/Connector/R2020b\"],\"version\":\"1.0\"}"
  "TT&C " : Subsystem
      settings: PortSchema="{\"entries\":[{\"content\":{\"headerSize\":26,\"margin\":15,\"minimumSpacing\":25,\"sides\":[{\"content\":{\"connectorIds\":[\"In1\"]},\"type\":\"ConnectorPlacement.EquallySpacedRectSide\",\"uuid\":\"e9a48b2f-fbc4-402d-8d97-df232b09ca74\"},{\"content\":{\"connectorIds\":[\"Out3\",\"Out2\"],\"side\":\"RIGHT\"},\"type\":\"ConnectorPlacement.EquallySpacedRectSide\",\"uuid\":\"668a9a5e-c59a-482e-88a8-af4c8ec5a9f3\"},{\"content\":{\"connectorIds\":[\"In2\"],\"side\":\"TOP\"},\"type\":\"ConnectorPlacement.EquallySpacedRectSide\",\"uuid\":\"7c7fce8b-f648-49b4-9dc1-b61d0240baf7\"},{\"content\":{\"connectorIds\":[\"In3\",\"Out1\"],\"side\":\"BOTTOM\"},\"type\":\"ConnectorPlacement.EquallySpacedRectSide\",\"uuid\":\"48187e99-04ba-46d1-bed4-4c5e9e3f3fd7\"}]},\"type\":\"ConnectorPlacement.EquallySpacedConnector\",\"uuid\":\"1f193ebe-c506-4262-ad28-c863fe0100e9\"}],\"packageUris\":[\"http://schema.mathworks.com/mf0/Connector/R2020b\"],\"version\":\"1.0\"}"
  Tether : Subsystem
      settings: PortSchema="{\"entries\":[{\"content\":{\"headerSize\":26,\"margin\":15,\"minimumSpacing\":25,\"sides\":[{\"content\":{\"connectorIds\":[\"LConn1\",\"LConn2\"]},\"type\":\"ConnectorPlacement.EquallySpacedRectSide\",\"uuid\":\"b0f3186e-f576-4647-b1a2-44485358b727\"},{\"content\":{\"connectorIds\":[\"In2\",\"In4\",\"In1\",\"Out2\"],\"side\":\"RIGHT\"},\"type\":\"ConnectorPlacement.EquallySpacedRectSide\",\"uuid\":\"71064ded-3aa0-4a06-beed-3d1d2c210288\"},{\"content\":{\"connectorIds\":[\"In3\",\"Out1\"],\"side\":\"TOP\"},\"type\":\"ConnectorPlacement.EquallySpacedRectSide\",\"uuid\":\"7b8a25e8-1259-40c4-b5f8-7d1b8fa69d47\"},{\"content\":{\"connectorIds\":[],\"side\":\"BOTTOM\"},\"type\":\"ConnectorPlacement.EquallySpacedRectSide\",\"uuid\":\"d0135317-6b67-4b35-89e9-958dc5eb3e20\"}]},\"type\":\"ConnectorPlacement.EquallySpacedConnector\",\"uuid\":\"e60708fb-7212-4361-80b1-30af05aaea9b\"}],\"packageUris\":[\"http://schema.mathworks.com/mf0/Connector/R2020b\"],\"version\":\"1.0\"}"
  TetherWire : PMIOPort  Side=Left
  Spring : PMIOPort  Port=2  Side=Left
  Bus Element Out4 : Outport  PortName=Telemetry B-G
  Bus Element Out3 : Outport  Port=2  PortName=ACK
  Bus Element Out2 : Outport  Port=3  PortName=Magnetorquers_Moment
  Bus Element Out1 : Outport  Port=4  PortName=Telemetray B-A
  wires:
  ADCS/2(Sensors_Data) -> OBC/5(Sensors_Data)
  EPS/6(EPS-Temp) -> TCS/1(EPS-Temp)
  EPS/8(OBC-Power) -> OBC/6(OBC-Power)
  EPS/9(TT&C-Power) -> "TT&C "/3(TT&C-Power)
  EPS/4(TCS-Power) -> TCS/2(TCS-Power)
  EPS/7(ADCS-Power) -> ADCS/2(ADCS-Power)
  Tether/1(Cam_data) -> OBC/4(Cam_data)
  OBC/5(Motor_Data) -> Tether/3(Motor_Data)
  EPS/3(Motor_Power) -> Tether/4(Motor_Power)
  Tether/2(PG_Power) -> EPS/2(PG_Power)
  EPS/5(ThS_Power) -> Tether/1(ThS_Power)
  EPS/1(Camera_Power) -> Tether/2(Camera_Power)
  "TT&C "/3(Command) -> OBC/3(Command)
  Bus Element In2/1 -> "TT&C "/2(Telecommand A-B)
  OBC/4(EPs_Switch_Command) -> EPS/1(EPs_Switch_Command)
  "TT&C "/1(ACK) -> Bus Element Out3/1
  EPS/2(PCDU_Data) -> OBC/2(PCDU_Data)
  "TT&C "/2(TTC_Data) -> OBC/1(TTC_Data)
  OBC/3(Telemetray B-A) -> Bus Element Out1/1
  ADCS/1(Magnetorquers_Moment) -> Bus Element Out2/1
  Bus Element In4/1 -> "TT&C "/1(Telecommand G-B)
  OBC/2(Telemetry B-G) -> Bus Element Out4/1
  OBC/1(OutBus) -> ADCS/1(InBus)
  connections:
  Tether/LConn1 -- TetherWire/RConn1
  Spring/RConn1 -- Tether/LConn2

== system SPARCS_Mission_System_Composer/End-body/Collector ==

== system SPARCS_Mission_System_Composer/End-body/Emitter ==

== system SPARCS_Mission_System_Composer/Environment/Atmosphere ==

== system SPARCS_Mission_System_Composer/Environment/Earth ==
  Magnetic Field : Subsystem  RequirementInfo={} %GIDa_33d46f3b_ea99_4103_948e_1808a1424f50
      settings: PortSchema="{\"entries\":[{\"content\":{\"headerSize\":26,\"margin\":15,\"minimumSpacing\":25,\"sides\":[{\"content\":{\"connectorIds\":[]},\"type\":\"ConnectorPlacement.EquallySpacedRectSide\",\"uuid\":\"a0205618-f388-4a93-9aec-aa689e4ebd78\"},{\"content\":{\"connectorIds\":[],\"side\":\"RIGHT\"},\"type\":\"ConnectorPlacement.EquallySpacedRectSide\",\"uuid\":\"79acb52b-c683-45c4-8f19-6aa7b44b6a95\"},{\"content\":{\"connectorIds\":[],\"side\":\"TOP\"},\"type\":\"ConnectorPlacement.EquallySpacedRectSide\",\"uuid\":\"1a3a54da-b4f5-4a0e-9102-49590a789f5c\"}]},\"type\":\"ConnectorPlacement.EquallySpacedConnector\",\"uuid\":\"e5b731ae-b390-48dd-b7a1-3459e2e6bab0\"}],\"packageUris\":[\"http://schema.mathworks.com/mf0/Connector/R2020b\"],\"version\":\"1.0\"}"

== system SPARCS_Mission_System_Composer/Environment/Sun ==
  Sun Vector : Subsystem  RequirementInfo={} %GIDa_25a3332d_e361_4ec4_8d1c_c7a7989470d3
      settings: PortSchema="{\"entries\":[{\"content\":{\"headerSize\":26,\"margin\":15,\"minimumSpacing\":25,\"sides\":[{\"content\":{\"connectorIds\":[]},\"type\":\"ConnectorPlacement.EquallySpacedRectSide\",\"uuid\":\"a0205618-f388-4a93-9aec-aa689e4ebd78\"},{\"content\":{\"connectorIds\":[],\"side\":\"RIGHT\"},\"type\":\"ConnectorPlacement.EquallySpacedRectSide\",\"uuid\":\"79acb52b-c683-45c4-8f19-6aa7b44b6a95\"},{\"content\":{\"connectorIds\":[],\"side\":\"TOP\"},\"type\":\"ConnectorPlacement.EquallySpacedRectSide\",\"uuid\":\"1a3a54da-b4f5-4a0e-9102-49590a789f5c\"}]},\"type\":\"ConnectorPlacement.EquallySpacedConnector\",\"uuid\":\"e5b731ae-b390-48dd-b7a1-3459e2e6bab0\"}],\"packageUris\":[\"http://schema.mathworks.com/mf0/Connector/R2020b\"],\"version\":\"1.0\"}"

== system SPARCS_Mission_System_Composer/Environment/Time ==

== system SPARCS_Mission_System_Composer/GS/Antenna Control Systems ==
  Bus Element In1 : Inport  RequirementInfo={} %GIDa_0ed5f7ca_a257_4aa9_9ea6_13af30c12930  PortName=AntennasPointingCommand
  Bus Element Out1 : Outport  RequirementInfo={} %GIDa_78e13a91_09d1_4043_b4f8_99a945310e74  PortName=AntennasPointing

== system SPARCS_Mission_System_Composer/GS/Antennas ==
  Bus Element In3 : Inport  RequirementInfo={} %GIDa_af5fb6c2_65b9_48c7_af1d_2c5f04b0ab86  PortName=TelecommadsData
  Bus Element In2 : Inport  RequirementInfo={} %GIDa_6138db1f_157a_44e3_a3b8_e7cea381d346  Port=2  PortName=AntennasPointing
  Bus Element In1 : Inport  RequirementInfo={} %GIDa_fe897c6a_03c0_4c94_a172_ef7dd5cfb766  Port=3  PortName=Telemetry
  Bus Element Out2 : Outport  RequirementInfo={} %GIDa_5a6ec1dd_67dd_48b7_8695_820321044ef9  PortName=TelemetryData
  Bus Element Out1 : Outport  RequirementInfo={} %GIDa_d2d7a6d1_77c4_4f26_a978_91bfd080235f  Port=2  PortName=Telecommand

== system SPARCS_Mission_System_Composer/GS/GS Station ==
  Bus Element In3 : Inport  RequirementInfo={} %GIDa_cc133ea9_9263_4158_9800_8c39fb3ae406  PortName=Order
  Bus Element In2 : Inport  RequirementInfo={} %GIDa_5541368e_c22e_42ea_a8c5_4fc13e90451f  Port=2  PortName=EnvGS
  Bus Element In1 : Inport  RequirementInfo={} %GIDa_0a0a1516_5b81_442a_bc4f_e18e6c73d98b  Port=3  PortName=TelemetryData
  Bus Element Out2 : Outport  RequirementInfo={} %GIDa_5832d44a_3382_48be_9ef2_96ec715fe740  PortName=TelecommadsData
  Bus Element Out1 : Outport  RequirementInfo={} %GIDa_9ae6d544_589e_47e8_8f3d_59c298361326  Port=2  PortName=AntennasPointingCommand

== system SPARCS_Mission_System_Composer/Launch System/Component ==

== system SPARCS_Mission_System_Composer/SPARCS-A/ADCS ==
  Bus Element In1 : Inport  PortName=ADCS-Power
  Bus Element Out1 : Outport  PortName=Magnetorquers_Moment
  Bus Element Out2 : Outport  Port=2  PortName=Sensors_Data

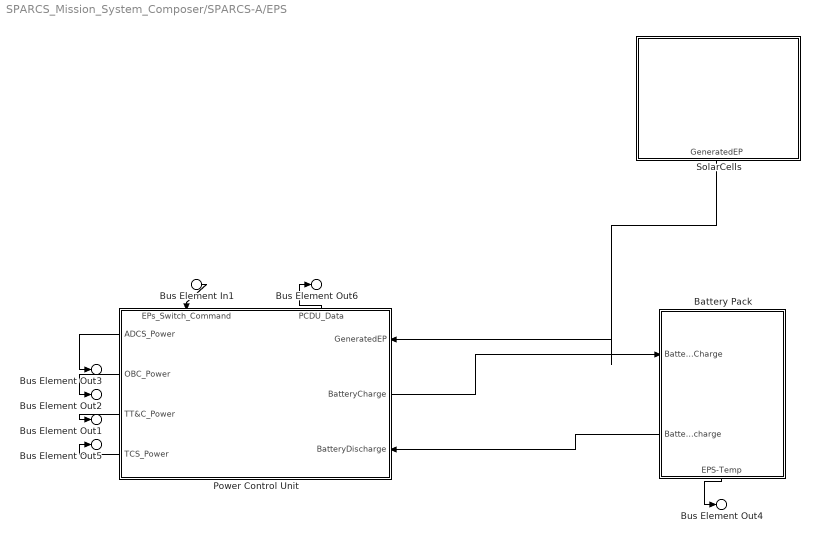
== system SPARCS_Mission_System_Composer/SPARCS-A/EPS ==
  Bus Element In1 : Inport  PortName=EPs_Switch_Command
  Battery Pack : Subsystem
      settings: PortSchema="{\"entries\":[{\"content\":{\"headerSize\":26,\"margin\":15,\"minimumSpacing\":25,\"sides\":[{\"content\":{\"connectorIds\":[\"In1\",\"Out2\"]},\"type\":\"ConnectorPlacement.EquallySpacedRectSide\",\"uuid\":\"a0205618-f388-4a93-9aec-aa689e4ebd78\"},{\"content\":{\"connectorIds\":[],\"side\":\"RIGHT\"},\"type\":\"ConnectorPlacement.EquallySpacedRectSide\",\"uuid\":\"79acb52b-c683-45c4-8f19-6aa7b44b6a95\"},{\"content\":{\"connectorIds\":[],\"side\":\"TOP\"},\"type\":\"ConnectorPlacement.EquallySpacedRectSide\",\"uuid\":\"1a3a54da-b4f5-4a0e-9102-49590a789f5c\"},{\"content\":{\"connectorIds\":[\"Out1\"],\"side\":\"BOTTOM\"},\"type\":\"ConnectorPlacement.EquallySpacedRectSide\",\"uuid\":\"779e32a4-6f4c-462e-a89d-e70261c77b0d\"}]},\"type\":\"ConnectorPlacement.EquallySpacedConnector\",\"uuid\":\"e5b731ae-b390-48dd-b7a1-3459e2e6bab0\"}],\"packageUris\":[\"http://schema.mathworks.com/mf0/Connector/R2020b\"],\"version\":\"1.0\"}"
  Power Control Unit : Subsystem
      settings: PortSchema="{\"entries\":[{\"content\":{\"headerSize\":26,\"margin\":15,\"minimumSpacing\":25,\"sides\":[{\"content\":{\"connectorIds\":[\"Out4\",\"Out5\",\"Out3\",\"Out2\"]},\"type\":\"ConnectorPlacement.EquallySpacedRectSide\",\"uuid\":\"a0205618-f388-4a93-9aec-aa689e4ebd78\"},{\"content\":{\"connectorIds\":[\"In1\",\"Out6\",\"In3\"],\"side\":\"RIGHT\"},\"type\":\"ConnectorPlacement.EquallySpacedRectSide\",\"uuid\":\"79acb52b-c683-45c4-8f19-6aa7b44b6a95\"},{\"content\":{\"connectorIds\":[\"In2\",\"Out1\"],\"side\":\"TOP\"},\"type\":\"ConnectorPlacement.EquallySpacedRectSide\",\"uuid\":\"1a3a54da-b4f5-4a0e-9102-49590a789f5c\"},{\"content\":{\"connectorIds\":[],\"side\":\"BOTTOM\"},\"type\":\"ConnectorPlacement.EquallySpacedRectSide\",\"uuid\":\"9b95dc80-80e8-43e3-a13a-4146a26c5b21\"}]},\"type\":\"ConnectorPlacement.EquallySpacedConnector\",\"uuid\":\"e5b731ae-b390-48dd-b7a1-3459e2e6bab0\"}],\"packageUris\":[\"http://schema.mathworks.com/mf0/Connector/R2020b\"],\"version\":\"1.0\"}"
  SolarCells : Subsystem
      settings: PortSchema="{\"entries\":[{\"content\":{\"headerSize\":26,\"margin\":15,\"minimumSpacing\":25,\"sides\":[{\"content\":{\"connectorIds\":[]},\"type\":\"ConnectorPlacement.EquallySpacedRectSide\",\"uuid\":\"a0205618-f388-4a93-9aec-aa689e4ebd78\"},{\"content\":{\"connectorIds\":[],\"side\":\"RIGHT\"},\"type\":\"ConnectorPlacement.EquallySpacedRectSide\",\"uuid\":\"79acb52b-c683-45c4-8f19-6aa7b44b6a95\"},{\"content\":{\"connectorIds\":[],\"side\":\"TOP\"},\"type\":\"ConnectorPlacement.EquallySpacedRectSide\",\"uuid\":\"1a3a54da-b4f5-4a0e-9102-49590a789f5c\"},{\"content\":{\"connectorIds\":[\"Out1\"],\"side\":\"BOTTOM\"},\"type\":\"ConnectorPlacement.EquallySpacedRectSide\",\"uuid\":\"0fe63fa1-99e2-42a9-86c7-5b07bc6faf14\"}]},\"type\":\"ConnectorPlacement.EquallySpacedConnector\",\"uuid\":\"e5b731ae-b390-48dd-b7a1-3459e2e6bab0\"}],\"packageUris\":[\"http://schema.mathworks.com/mf0/Connector/R2020b\"],\"version\":\"1.0\"}"
  Bus Element Out6 : Outport  PortName=PCDU_Data
  Bus Element Out5 : Outport  Port=2  PortName=TCS_Power
  Bus Element Out4 : Outport  Port=3  PortName=EPS-Temp
  Bus Element Out3 : Outport  Port=4  PortName=ADCS_Power
  Bus Element Out2 : Outport  Port=5  PortName=OBC_Power
  Bus Element Out1 : Outport  Port=6  PortName=TT&C_Power
  wires:
  Battery Pack/2(BatteryDischarge) -> Power Control Unit/3(BatteryDischarge)
  Power Control Unit/6(BatteryCharge) -> Battery Pack/1(BatteryCharge)
  SolarCells/1(GeneratedEP) -> Power Control Unit/1(GeneratedEP)
  Power Control Unit/4(ADCS_Power) -> Bus Element Out3/1
  Power Control Unit/5(OBC_Power) -> Bus Element Out2/1
  Power Control Unit/3(TT&C_Power) -> Bus Element Out1/1
  Power Control Unit/2(TCS_Power) -> Bus Element Out5/1
  Battery Pack/1(EPS-Temp) -> Bus Element Out4/1
  Power Control Unit/1(PCDU_Data) -> Bus Element Out6/1
  Bus Element In1/1 -> Power Control Unit/2(EPs_Switch_Command)

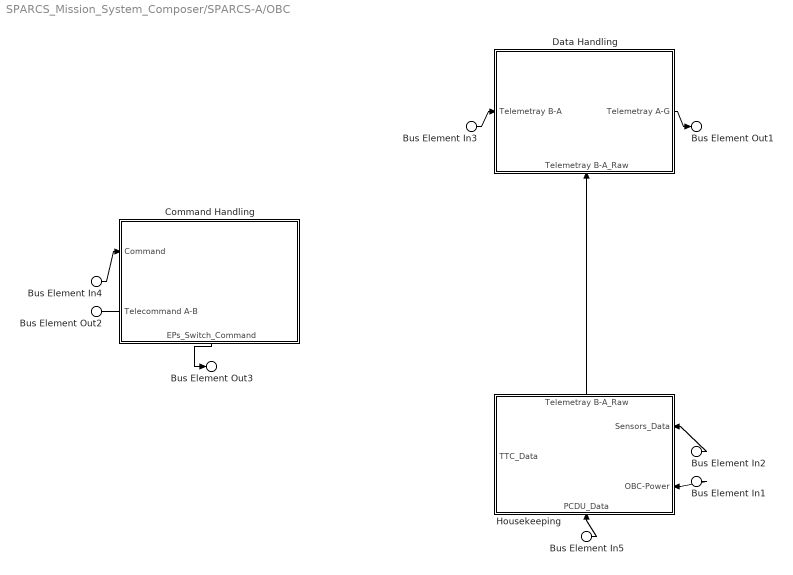
== system SPARCS_Mission_System_Composer/SPARCS-A/OBC ==
  Bus Element In4 : Inport  PortName=Command
  Bus Element In5 : Inport  Port=2  PortName=PCDU_Data
  Bus Element In3 : Inport  Port=3  PortName=Telemetray B-A
  Bus Element In2 : Inport  Port=4  PortName=Sensors_Data
  Bus Element In1 : Inport  Port=5  PortName=OBC-Power
  "Command Handling " : Subsystem
      settings: PortSchema="{\"entries\":[{\"content\":{\"headerSize\":26,\"margin\":15,\"minimumSpacing\":25,\"sides\":[{\"content\":{\"connectorIds\":[\"In1\",\"Out1\"]},\"type\":\"ConnectorPlacement.EquallySpacedRectSide\",\"uuid\":\"55446906-0beb-490e-966b-fd119ff7d790\"},{\"content\":{\"connectorIds\":[],\"side\":\"RIGHT\"},\"type\":\"ConnectorPlacement.EquallySpacedRectSide\",\"uuid\":\"4b5c9eb0-c92d-45b7-8098-5a0979f0d9fd\"},{\"content\":{\"connectorIds\":[],\"side\":\"TOP\"},\"type\":\"ConnectorPlacement.EquallySpacedRectSide\",\"uuid\":\"16aec1aa-8dc3-4431-a56b-4fb7824e2a96\"},{\"content\":{\"connectorIds\":[\"Out2\"],\"side\":\"BOTTOM\"},\"type\":\"ConnectorPlacement.EquallySpacedRectSide\",\"uuid\":\"6e384acb-5329-47af-a18c-2030ef64aa13\"}]},\"type\":\"ConnectorPlacement.EquallySpacedConnector\",\"uuid\":\"1865971b-538c-48f2-a7a3-1f3aa40ff883\"}],\"packageUris\":[\"http://schema.mathworks.com/mf0/Connector/R2020b\"],\"version\":\"1.0\"}"
  "Data Handling " : Subsystem
      settings: PortSchema="{\"entries\":[{\"content\":{\"headerSize\":26,\"margin\":15,\"minimumSpacing\":25,\"sides\":[{\"content\":{\"connectorIds\":[\"In1\"]},\"type\":\"ConnectorPlacement.EquallySpacedRectSide\",\"uuid\":\"55446906-0beb-490e-966b-fd119ff7d790\"},{\"content\":{\"connectorIds\":[\"Out1\"],\"side\":\"RIGHT\"},\"type\":\"ConnectorPlacement.EquallySpacedRectSide\",\"uuid\":\"4b5c9eb0-c92d-45b7-8098-5a0979f0d9fd\"},{\"content\":{\"connectorIds\":[],\"side\":\"TOP\"},\"type\":\"ConnectorPlacement.EquallySpacedRectSide\",\"uuid\":\"16aec1aa-8dc3-4431-a56b-4fb7824e2a96\"},{\"content\":{\"connectorIds\":[\"In2\"],\"side\":\"BOTTOM\"},\"type\":\"ConnectorPlacement.EquallySpacedRectSide\",\"uuid\":\"1a5ced55-66af-4bf0-87a3-c6b9f0175afd\"}]},\"type\":\"ConnectorPlacement.EquallySpacedConnector\",\"uuid\":\"1865971b-538c-48f2-a7a3-1f3aa40ff883\"}],\"packageUris\":[\"http://schema.mathworks.com/mf0/Connector/R2020b\"],\"version\":\"1.0\"}"
  Housekeeping : Subsystem
      settings: PortSchema="{\"entries\":[{\"content\":{\"headerSize\":26,\"margin\":15,\"minimumSpacing\":25,\"sides\":[{\"content\":{\"connectorIds\":[\"In3\"]},\"type\":\"ConnectorPlacement.EquallySpacedRectSide\",\"uuid\":\"55446906-0beb-490e-966b-fd119ff7d790\"},{\"content\":{\"connectorIds\":[\"In1\",\"In2\"],\"side\":\"RIGHT\"},\"type\":\"ConnectorPlacement.EquallySpacedRectSide\",\"uuid\":\"4b5c9eb0-c92d-45b7-8098-5a0979f0d9fd\"},{\"content\":{\"connectorIds\":[\"Out1\"],\"side\":\"TOP\"},\"type\":\"ConnectorPlacement.EquallySpacedRectSide\",\"uuid\":\"16aec1aa-8dc3-4431-a56b-4fb7824e2a96\"},{\"content\":{\"connectorIds\":[\"In4\"],\"side\":\"BOTTOM\"},\"type\":\"ConnectorPlacement.EquallySpacedRectSide\",\"uuid\":\"92354330-e6e6-44e5-aa17-e05d5ad5204a\"}]},\"type\":\"ConnectorPlacement.EquallySpacedConnector\",\"uuid\":\"1865971b-538c-48f2-a7a3-1f3aa40ff883\"}],\"packageUris\":[\"http://schema.mathworks.com/mf0/Connector/R2020b\"],\"version\":\"1.0\"}"
  Bus Element Out3 : Outport  PortName=EPs_Switch_Command
  Bus Element Out2 : Outport  Port=2  PortName=Telecommand A-B
  Bus Element Out1 : Outport  Port=3  PortName=Telemetray A-G
  wires:
  Bus Element In4/1 -> "Command Handling "/1(Command)
  "Command Handling "/1(Telecommand A-B) -> Bus Element Out2/1
  Bus Element In1/1 -> Housekeeping/2(OBC-Power)
  Bus Element In2/1 -> Housekeeping/1(Sensors_Data)
  Bus Element In3/1 -> "Data Handling "/1(Telemetray B-A)
  Bus Element In5/1 -> Housekeeping/4(PCDU_Data)
  "Command Handling "/2(EPs_Switch_Command) -> Bus Element Out3/1
  Housekeeping/1(Telemetray B-A_Raw) -> "Data Handling "/2(Telemetray B-A_Raw)
  "Data Handling "/1(Telemetray A-G) -> Bus Element Out1/1

== system SPARCS_Mission_System_Composer/SPARCS-A/TCS ==
  Bus Element In2 : Inport  PortName=EPS-Temp
  Bus Element In1 : Inport  Port=2  PortName=TCS-Power

== system SPARCS_Mission_System_Composer/SPARCS-A/TT&C  ==
  Bus Element In3 : Inport  PortName=ACK
  Bus Element In2 : Inport  Port=2  PortName=Telecommand G-A
  Bus Element In1 : Inport  Port=3  PortName=TT&C-Power
  Antennas : Subsystem
      settings: PortSchema="{\"entries\":[{\"content\":{\"headerSize\":26,\"margin\":15,\"minimumSpacing\":25,\"sides\":[{\"content\":{\"connectorIds\":[]},\"type\":\"ConnectorPlacement.EquallySpacedRectSide\",\"uuid\":\"b8e64c0e-f241-43e7-badf-308c180049c9\"},{\"content\":{\"connectorIds\":[],\"side\":\"RIGHT\"},\"type\":\"ConnectorPlacement.EquallySpacedRectSide\",\"uuid\":\"146de698-4586-43ed-80a1-9a25d4f72af0\"},{\"content\":{\"connectorIds\":[],\"side\":\"TOP\"},\"type\":\"ConnectorPlacement.EquallySpacedRectSide\",\"uuid\":\"022d51e1-8d8c-4400-9819-a59e0bf78e40\"}]},\"type\":\"ConnectorPlacement.EquallySpacedConnector\",\"uuid\":\"3d3eda84-2dfa-49ef-a4f2-f7a393d07487\"}],\"packageUris\":[\"http://schema.mathworks.com/mf0/Connector/R2020b\"],\"version\":\"1.0\"}"
  ISL : Subsystem
      settings: PortSchema="{\"entries\":[{\"content\":{\"headerSize\":26,\"margin\":15,\"minimumSpacing\":25,\"sides\":[{\"content\":{\"connectorIds\":[]},\"type\":\"ConnectorPlacement.EquallySpacedRectSide\",\"uuid\":\"55446906-0beb-490e-966b-fd119ff7d790\"},{\"content\":{\"connectorIds\":[],\"side\":\"RIGHT\"},\"type\":\"ConnectorPlacement.EquallySpacedRectSide\",\"uuid\":\"4b5c9eb0-c92d-45b7-8098-5a0979f0d9fd\"},{\"content\":{\"connectorIds\":[\"Out1\"],\"side\":\"TOP\"},\"type\":\"ConnectorPlacement.EquallySpacedRectSide\",\"uuid\":\"16aec1aa-8dc3-4431-a56b-4fb7824e2a96\"},{\"content\":{\"connectorIds\":[\"In1\"],\"side\":\"BOTTOM\"},\"type\":\"ConnectorPlacement.EquallySpacedRectSide\",\"uuid\":\"431945b6-1943-47a1-8f54-a0360a38c518\"}]},\"type\":\"ConnectorPlacement.EquallySpacedConnector\",\"uuid\":\"1865971b-538c-48f2-a7a3-1f3aa40ff883\"}],\"packageUris\":[\"http://schema.mathworks.com/mf0/Connector/R2020b\"],\"version\":\"1.0\"}"
  TT&C Board : Subsystem
      settings: PortSchema="{\"entries\":[{\"content\":{\"headerSize\":26,\"margin\":15,\"minimumSpacing\":25,\"sides\":[{\"content\":{\"connectorIds\":[]},\"type\":\"ConnectorPlacement.EquallySpacedRectSide\",\"uuid\":\"b8e64c0e-f241-43e7-badf-308c180049c9\"},{\"content\":{\"connectorIds\":[],\"side\":\"RIGHT\"},\"type\":\"ConnectorPlacement.EquallySpacedRectSide\",\"uuid\":\"146de698-4586-43ed-80a1-9a25d4f72af0\"},{\"content\":{\"connectorIds\":[],\"side\":\"TOP\"},\"type\":\"ConnectorPlacement.EquallySpacedRectSide\",\"uuid\":\"022d51e1-8d8c-4400-9819-a59e0bf78e40\"}]},\"type\":\"ConnectorPlacement.EquallySpacedConnector\",\"uuid\":\"3d3eda84-2dfa-49ef-a4f2-f7a393d07487\"}],\"packageUris\":[\"http://schema.mathworks.com/mf0/Connector/R2020b\"],\"version\":\"1.0\"}"
  Bus Element Out1 : Outport  PortName=Command
  wires:
  Bus Element In3/1 -> ISL/1(ACK)
  ISL/1(Command) -> Bus Element Out1/1

== system SPARCS_Mission_System_Composer/SPARCS-B/ADCS ==
  Bus Element In2 : Inport  PortName=InBus
  Bus Element In1 : Inport  Port=2  PortName=ADCS-Power
  Bus Element Out1 : Outport  PortName=Magnetorquers_Moment
  Bus Element Out2 : Outport  Port=2  PortName=Sensors_Data
